simulink model "lab1"  (R2017a)
settings: Solver=VariableStepAuto  StartTime=0.0  StopTime=16.00  RelTol=1e-3
libraries: dspsrcs4 x1, dspxfrm3 x1
settings Model: Creator=yurij  LastModifiedBy=yurij

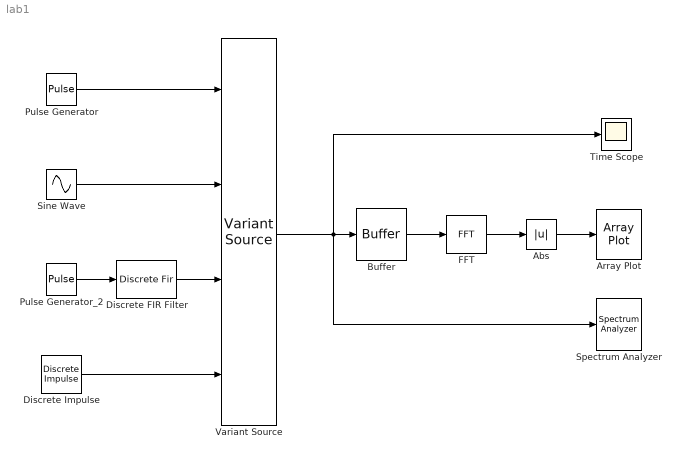
== system lab1 ==
  Abs : Abs
  Array Plot : ArrayPlot
  Buffer : Buffer  N=1024  OutputFrames=off
  Discrete Impulse : dspsrcs4/Discrete  Impulse  Delay=0:100:1600  SampleTime=0.01  FrameSample=10  OutputFrames=off  dataType=double  isSigned=on  wordLen=16  udDataType=sfix(16)  fracBitsMode=Best precision  numFracBits=15  OutDataTypeStr=double  LastOutDataTypeStr=double
  Discrete FIR Filter : DiscreteFir  Coefficients=ones(1, 50) / 50
  FFT : dspxfrm3/FFT  FFTImplementation=Auto  CompMethod=Table lookup  TableOpt=NEW  TableOptActive=Speed  BitRevOrder=off  Normalize=off  InheritFFTLength=on  FFTLength=64  WrapInput=on  roundingMode=Floor  overflowMode=off  firstCoeffDataTypeStr=Inherit: Same word length as input  firstCoeffLastDataTypeStr=Inherit: Same word length as input  outputMin=[]  outputMax=[]
  Pulse Generator : DiscretePulseGenerator  Period=100  PulseWidth=50  SampleTime=0.01
  "Pulse Generator_2 " : DiscretePulseGenerator  Period=100  PulseWidth=50  SampleTime=0.01
  Sine Wave : Sin  Frequency=3  SampleTime=0.01
  Spectrum Analyzer : SpectrumAnalyzer
  Time Scope : Scope
  Variant Source : VariantSource  OverrideUsingVariant=S==2  ShowConditionOnBlock=on
  wires:
  Variant Source/1 -> Spectrum Analyzer/1, Buffer/1, Time Scope/1
  Buffer/1 -> FFT/1
  Abs/1 -> Array Plot/1
  FFT/1 -> Abs/1
  Pulse Generator/1 -> Variant Source/1
  Sine Wave/1 -> Variant Source/2
  "Pulse Generator_2 "/1 -> Discrete FIR Filter/1
  Discrete FIR Filter/1 -> Variant Source/3
  Discrete Impulse/1 -> Variant Source/4
